simulink model "wah"  (R2025b)
settings: Solver=FixedStepDiscrete  StartTime=0.0  StopTime=inf  RelTol=1e-3
undefined symbols (not defined in the file or in its folder): Depth_rt, FilterGain_rt, Fmax_rt, Fmin_rt, Gain_rt, iPhase_rt, Q_rt, Rate_rt, Type_rt, WaveSel_rt
settings Model: Creator=linogarciamorales  LastModifiedBy=linogarciamorales
settings OptimizationCC: EnhancedBackFolding=on  PassReuseOutputArgsAs=Individual arguments  ZeroExternalMemoryAtStartup=off  ZeroInternalMemoryAtStartup=off  OptimizeBlockOrder=speed  DifferentSizesBufferReuse=on  OptimizationCustomize=off  EfficientTunableParamExpr=on
settings DebuggingCC: ParameterTunabilityLossMsg=error
settings HardwareCC: ProdBitPerPointer=32.0  ProdBitPerSizeT=32.0  ProdBitPerPtrDiffT=32.0  ProdLargestAtomicFloat=None  ProdIntDivRoundTo=Undefined  ProdEndianess=Unspecified  ProdWordSize=32.0  ProdHWDeviceType=Generic->32-bit Embedded Processor
settings SFSimCC: MATLABDynamicMemAlloc=off
settings RTWCC: SystemTargetFile=ert.tlc  GenCodeOnly=on  TemplateMakefile=ert_default_tmf  Description=Embedded Coder
settings CodeAppCC: ForceParamTrailComments=on  IgnoreCustomStorageClasses=off  OperatorAnnotations=on  SimulinkDataObjDesc=on  SFDataObjDesc=on  InsertBlockDesc=on
settings ERTTargetCC: InlinedParameterPlacement=Hierarchical  ERTCustomFileTemplate=example_file_process.tlc  TargetLangStandard=C99 (ISO)  SupportNonInlinedSFcns=on

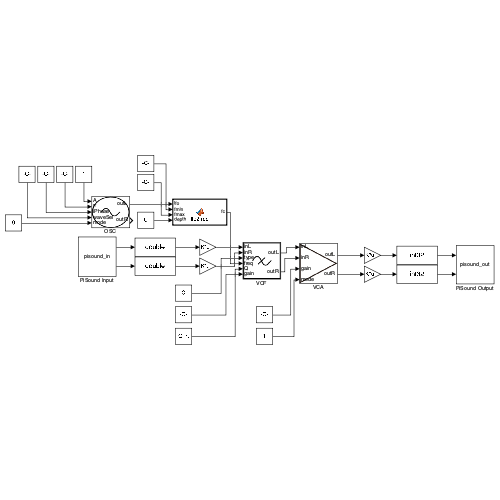
[thumbnail: Simulink's stored preview of the top-level diagram]
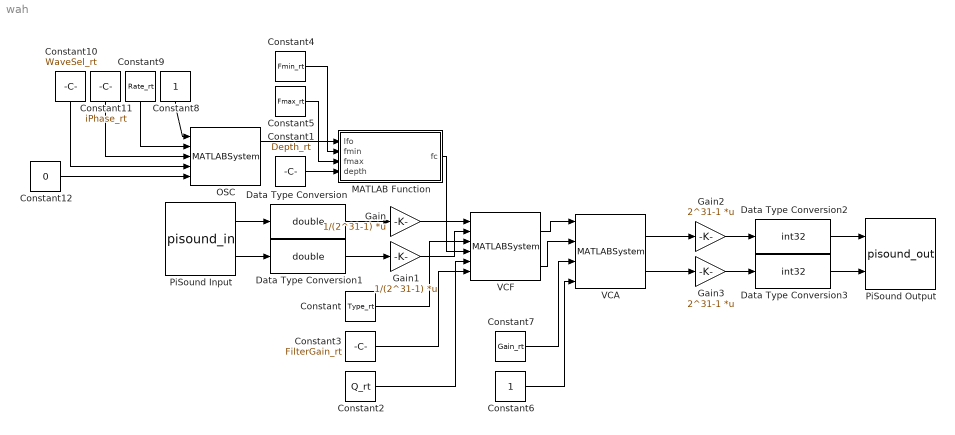
== system wah ==
  Constant : Constant  Value=Type_rt  OutDataTypeStr=uint8
  Constant1 : Constant  Value=Depth_rt  OutDataTypeStr=double
  Constant10 : Constant  Value=WaveSel_rt  OutDataTypeStr=uint8
  Constant11 : Constant  Value=iPhase_rt  OutDataTypeStr=double
  Constant12 : Constant  Value=0  OutDataTypeStr=uint8
  Constant2 : Constant  Value=Q_rt  OutDataTypeStr=double
  Constant3 : Constant  Value=FilterGain_rt  OutDataTypeStr=double
  Constant4 : Constant  Value=Fmin_rt
  Constant5 : Constant  Value=Fmax_rt
  Constant6 : Constant  OutDataTypeStr=uint8
  Constant7 : Constant  Value=Gain_rt  OutDataTypeStr=double
  Constant8 : Constant  OutDataTypeStr=double
  Constant9 : Constant  Value=Rate_rt  OutDataTypeStr=double
  Data Type Conversion : DataTypeConversion  OutDataTypeStr=double  SaturateOnIntegerOverflow=off  RndMeth=Floor
  Data Type Conversion1 : DataTypeConversion  OutDataTypeStr=double  SaturateOnIntegerOverflow=off  RndMeth=Floor
  Data Type Conversion2 : DataTypeConversion  OutDataTypeStr=int32  SaturateOnIntegerOverflow=off  RndMeth=Floor
  Data Type Conversion3 : DataTypeConversion  OutDataTypeStr=int32  SaturateOnIntegerOverflow=off  RndMeth=Floor
  Gain : Gain  Gain=1/(2^31-1)  Multiplication=Matrix(K*u)
  Gain1 : Gain  Gain=1/(2^31-1)  Multiplication=Matrix(K*u)
  Gain2 : Gain  Gain=2^31-1  Multiplication=Matrix(K*u)
  Gain3 : Gain  Gain=2^31-1  Multiplication=Matrix(K*u)
  MATLAB Function : MATLAB Function  TreatAsAtomicUnit=on
  OSC : MATLABSystem  System=vco_sys  N=128  Fs=48000  OutMaxL=4096  InFixL=1024  SimulateUsing=Code generation
      mask Type: vco_sys
  PiSound Input : S-Function  FunctionName=pisound_in  Parameters=48000, 128, 0  SFunctionDeploymentMode=off  EnableBusSupport=off
  PiSound Output : S-Function  FunctionName=pisound_out  Parameters=48000, 128, 0  SFunctionDeploymentMode=off  EnableBusSupport=off
  VCA : MATLABSystem  System=vca_sys  N=128  Fs=48000  bypass=uint8(0)  SimulateUsing=Code generation
      mask Type: vca_sys
  VCF : MATLABSystem  InitFcn=|  System=vcf_sys  N=128  Fs=48000  bypass=uint8(0)  SimulateUsing=Code generation
      | Type_rt = uint8(1);   % 1..7
      | Freq_rt = 1000;       % Hz
      | Q_rt    = 0.707;
      | Gain_rt = 0;          % dB
      mask Type: vcf_sys
  wires:
  PiSound Input/1 -> Data Type Conversion/1
  PiSound Input/2 -> Data Type Conversion1/1
  Data Type Conversion/1 -> Gain/1
  Data Type Conversion1/1 -> Gain1/1
  Gain2/1 -> Data Type Conversion2/1
  Gain3/1 -> Data Type Conversion3/1
  Data Type Conversion2/1 -> PiSound Output/1
  Data Type Conversion3/1 -> PiSound Output/2
  Constant2/1 -> VCF/5
  Constant3/1 -> VCF/6
  Constant4/1 -> MATLAB Function/2(fmin)
  OSC/1 -> MATLAB Function/1(lfo)
  Constant5/1 -> MATLAB Function/3(fmax)
  Constant/1 -> VCF/3
  Constant1/1 -> MATLAB Function/4(depth)
  Gain/1 -> VCF/1
  Gain1/1 -> VCF/2
  VCF/1 -> VCA/1
  MATLAB Function/1(fc) -> VCF/4
  VCA/1 -> Gain2/1
  VCA/2 -> Gain3/1
  VCF/2 -> VCA/2
  Constant6/1 -> VCA/4
  Constant7/1 -> VCA/3
  Constant8/1 -> OSC/1
  Constant9/1 -> OSC/2
  Constant10/1 -> OSC/4
  Constant11/1 -> OSC/3
  Constant12/1 -> OSC/5

== matlab function wah/MATLAB Function ==
  data: lfo input; fc output; fmin input; fmax input; depth input
function fc = lfo2freq(lfo,fmin,fmax,depth)
l = mean(double(lfo));                 % <- en vez de lfo(1)
l = max(-1,min(1,l));

fmin = double(fmin); fmax = double(fmax);
if fmax < fmin, tmp=fmin; fmin=fmax; fmax=tmp; end
if fmin <= 0, fmin = 0.1; end
if fmax <= fmin, fmax = fmin*2; end

depth = max(0,min(1,double(depth)));

f0 = sqrt(fmin*fmax);
R  = fmax/fmin;
fc = f0 * exp((log(R)/2)*(depth*l));
end
